simulink model "HW4_4"  (R2023a)
settings: Solver=VariableStepAuto  StartTime=0.0  StopTime=10.0  RelTol=1e-3
settings Model: Creator=BRL  LastModifiedBy=BRL

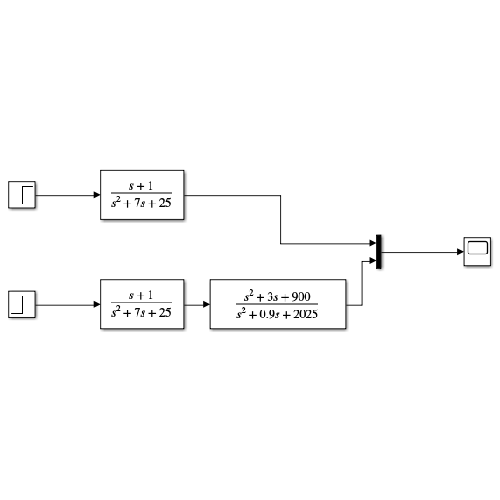
[thumbnail: Simulink's stored preview of the top-level diagram]
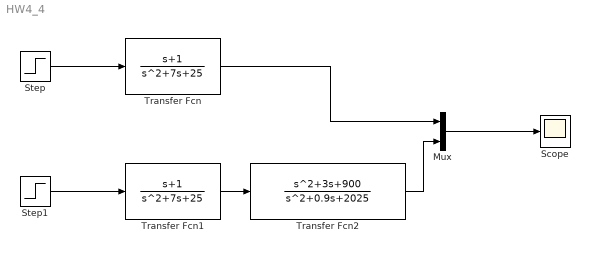
== system HW4_4 ==
  Mux : Mux  Inputs=2
  Scope : Scope
  Step : Step  SampleTime=0
  Step1 : Step  SampleTime=0
  Transfer Fcn : TransferFcn  Numerator=[1 1]  Denominator=[1 7 25]
  Transfer Fcn1 : TransferFcn  Numerator=[1 1]  Denominator=[1 7 25]
  Transfer Fcn2 : TransferFcn  Numerator=[1 3 900]  Denominator=[1 0.9 2025]
  wires:
  Step/1 -> Transfer Fcn/1
  Step1/1 -> Transfer Fcn1/1
  Mux/1 -> Scope/1
  Transfer Fcn2/1 -> Mux/2
  Transfer Fcn1/1 -> Transfer Fcn2/1
  Transfer Fcn/1 -> Mux/1
